simulink model "Ejercicio_2a"  (R2013a)
settings: Solver=ode45  StartTime=0.0  StopTime=10.0  RelTol=1e-3
settings Model: Creator=LuisFernando  LastModifiedBy=LuisFernando

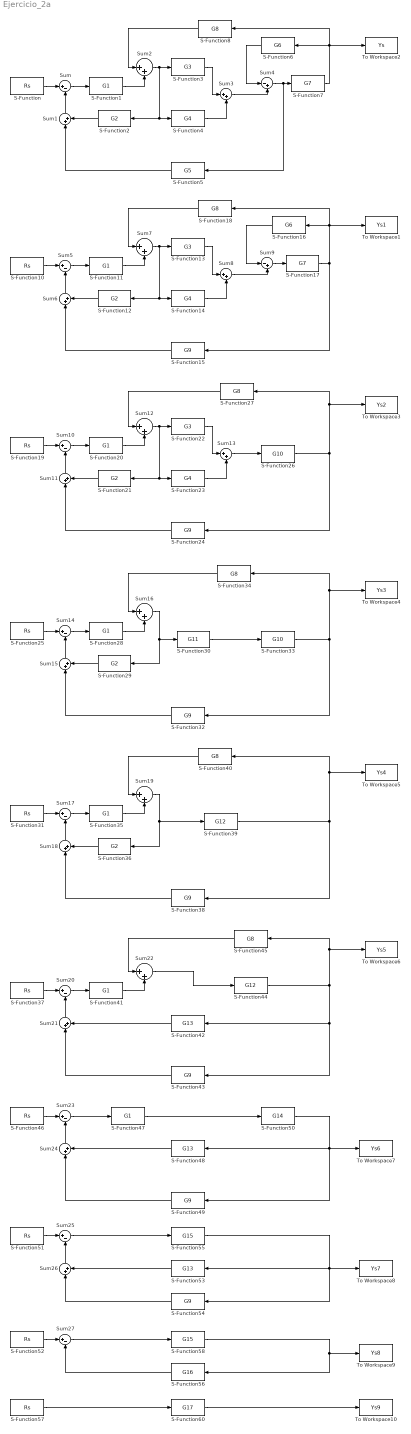
== system Ejercicio_2a ==
  S-Function{,10,19,25,31,37,46,51..52,57} (10 alike) : S-Function  FunctionName=Rs  EnableBusSupport=off
  S-Function{1,11,20,28,35,41,47} (7 alike) : S-Function  FunctionName=G1  EnableBusSupport=off
  S-Function{2,12,21,29,36} (5 alike) : S-Function  FunctionName=G2  EnableBusSupport=off
  S-Function13 : S-Function  FunctionName=G3  EnableBusSupport=off
  S-Function14 : S-Function  FunctionName=G4  EnableBusSupport=off
  S-Function{15,24,32,38,43,49,54} (7 alike) : S-Function  FunctionName=G9  EnableBusSupport=off
  S-Function16 : S-Function  FunctionName=G6  EnableBusSupport=off
  S-Function17 : S-Function  FunctionName=G7  EnableBusSupport=off
  S-Function{8,18,27,34,40,45} (6 alike) : S-Function  FunctionName=G8  EnableBusSupport=off
  S-Function22 : S-Function  FunctionName=G3  EnableBusSupport=off
  S-Function23 : S-Function  FunctionName=G4  EnableBusSupport=off
  S-Function26 : S-Function  FunctionName=G10  EnableBusSupport=off
  S-Function3 : S-Function  FunctionName=G3  EnableBusSupport=off
  S-Function30 : S-Function  FunctionName=G11  EnableBusSupport=off
  S-Function33 : S-Function  FunctionName=G10  EnableBusSupport=off
  S-Function39 : S-Function  FunctionName=G12  EnableBusSupport=off
  S-Function4 : S-Function  FunctionName=G4  EnableBusSupport=off
  S-Function42 : S-Function  FunctionName=G13  EnableBusSupport=off
  S-Function44 : S-Function  FunctionName=G12  EnableBusSupport=off
  S-Function48 : S-Function  FunctionName=G13  EnableBusSupport=off
  S-Function5 : S-Function  FunctionName=G5  EnableBusSupport=off
  S-Function50 : S-Function  FunctionName=G14  EnableBusSupport=off
  S-Function53 : S-Function  FunctionName=G13  EnableBusSupport=off
  S-Function55 : S-Function  FunctionName=G15  EnableBusSupport=off
  S-Function56 : S-Function  FunctionName=G16  EnableBusSupport=off
  S-Function58 : S-Function  FunctionName=G15  EnableBusSupport=off
  S-Function6 : S-Function  FunctionName=G6  EnableBusSupport=off
  S-Function60 : S-Function  FunctionName=G17  EnableBusSupport=off
  S-Function7 : S-Function  FunctionName=G7  EnableBusSupport=off
  Sum{,5,10,14,17,20,23,25,27} (9 alike) : Sum  Inputs=|+-
  Sum{1..3,6..8,11..13,15..16,18..19,21..22,24,26} (17 alike) : Sum  Inputs=|++
  Sum4 : Sum  Inputs=|-+
  Sum9 : Sum  Inputs=|-+
  To Workspace1 : ToWorkspace  VariableName=Ys1  SampleTime=-1
  To Workspace10 : ToWorkspace  VariableName=Ys9  SampleTime=-1
  To Workspace2 : ToWorkspace  VariableName=Ys  SampleTime=-1
  To Workspace3 : ToWorkspace  VariableName=Ys2  SampleTime=-1
  To Workspace4 : ToWorkspace  VariableName=Ys3  SampleTime=-1
  To Workspace5 : ToWorkspace  VariableName=Ys4  SampleTime=-1
  To Workspace6 : ToWorkspace  VariableName=Ys5  SampleTime=-1
  To Workspace7 : ToWorkspace  VariableName=Ys6  SampleTime=-1
  To Workspace8 : ToWorkspace  VariableName=Ys7  SampleTime=-1
  To Workspace9 : ToWorkspace  VariableName=Ys8  SampleTime=-1
  wires:
  S-Function8/1 -> Sum2/1
  S-Function1/1 -> Sum2/2
  Sum/1 -> S-Function1/1
  Sum1/1 -> Sum/2
  S-Function2/1 -> Sum1/2
  S-Function5/1 -> Sum1/1
  S-Function3/1 -> Sum3/1
  S-Function4/1 -> Sum3/2
  Sum3/1 -> Sum4/2
  S-Function6/1 -> Sum4/1
  Sum4/1 -> S-Function7/1, S-Function5/1
  S-Function7/1 -> S-Function8/1, S-Function6/1, To Workspace2/1
  Sum2/1 -> S-Function3/1, S-Function4/1, S-Function2/1
  S-Function/1 -> Sum/1
  S-Function18/1 -> Sum7/1
  S-Function11/1 -> Sum7/2
  Sum5/1 -> S-Function11/1
  Sum6/1 -> Sum5/2
  S-Function12/1 -> Sum6/2
  S-Function15/1 -> Sum6/1
  S-Function13/1 -> Sum8/1
  S-Function14/1 -> Sum8/2
  Sum8/1 -> Sum9/2
  S-Function16/1 -> Sum9/1
  Sum9/1 -> S-Function17/1
  S-Function17/1 -> S-Function18/1, S-Function16/1, To Workspace1/1, S-Function15/1
  Sum7/1 -> S-Function13/1, S-Function14/1, S-Function12/1
  S-Function10/1 -> Sum5/1
  S-Function27/1 -> Sum12/1
  S-Function20/1 -> Sum12/2
  Sum10/1 -> S-Function20/1
  Sum11/1 -> Sum10/2
  S-Function21/1 -> Sum11/2
  S-Function24/1 -> Sum11/1
  S-Function22/1 -> Sum13/1
  S-Function23/1 -> Sum13/2
  S-Function26/1 -> S-Function27/1, To Workspace3/1, S-Function24/1
  Sum12/1 -> S-Function22/1, S-Function23/1, S-Function21/1
  S-Function19/1 -> Sum10/1
  Sum13/1 -> S-Function26/1
  S-Function34/1 -> Sum16/1
  S-Function28/1 -> Sum16/2
  Sum14/1 -> S-Function28/1
  Sum15/1 -> Sum14/2
  S-Function29/1 -> Sum15/2
  S-Function32/1 -> Sum15/1
  S-Function33/1 -> S-Function34/1, To Workspace4/1, S-Function32/1
  Sum16/1 -> S-Function30/1, S-Function29/1
  S-Function25/1 -> Sum14/1
  S-Function30/1 -> S-Function33/1
  S-Function40/1 -> Sum19/1
  S-Function35/1 -> Sum19/2
  Sum17/1 -> S-Function35/1
  Sum18/1 -> Sum17/2
  S-Function36/1 -> Sum18/2
  S-Function38/1 -> Sum18/1
  S-Function39/1 -> S-Function40/1, To Workspace5/1, S-Function38/1
  Sum19/1 -> S-Function39/1, S-Function36/1
  S-Function31/1 -> Sum17/1
  S-Function45/1 -> Sum22/1
  S-Function41/1 -> Sum22/2
  Sum20/1 -> S-Function41/1
  Sum21/1 -> Sum20/2
  S-Function42/1 -> Sum21/2
  S-Function43/1 -> Sum21/1
  Sum22/1 -> S-Function44/1
  S-Function37/1 -> Sum20/1
  S-Function44/1 -> S-Function45/1, To Workspace6/1, S-Function42/1, S-Function43/1
  Sum23/1 -> S-Function47/1
  Sum24/1 -> Sum23/2
  S-Function48/1 -> Sum24/2
  S-Function49/1 -> Sum24/1
  S-Function46/1 -> Sum23/1
  S-Function50/1 -> To Workspace7/1, S-Function48/1, S-Function49/1
  S-Function47/1 -> S-Function50/1
  Sum26/1 -> Sum25/2
  S-Function53/1 -> Sum26/2
  S-Function54/1 -> Sum26/1
  S-Function51/1 -> Sum25/1
  S-Function55/1 -> To Workspace8/1, S-Function53/1, S-Function54/1
  Sum25/1 -> S-Function55/1
  S-Function52/1 -> Sum27/1
  S-Function58/1 -> S-Function56/1, To Workspace9/1
  Sum27/1 -> S-Function58/1
  S-Function56/1 -> Sum27/2
  S-Function60/1 -> To Workspace10/1
  S-Function57/1 -> S-Function60/1
